simulink model "IceWheel_ControlDesign_Simulink"  (R2021b)
settings: Solver=VariableStepAuto  StartTime=0.0  StopTime=8  RelTol=1e-3
undefined symbols (not defined in the file or in its folder): A, B, C, D, k_m, K_p, T_d, T_motor
libraries: slpidlib x1
settings Model: Creator=elias  LastModifiedBy=SwisensAG
settings SolverCC: AlgebraicLoopSolver=TrustRegion
settings DebuggingCC: SFMachineParentedDataDiag=warning

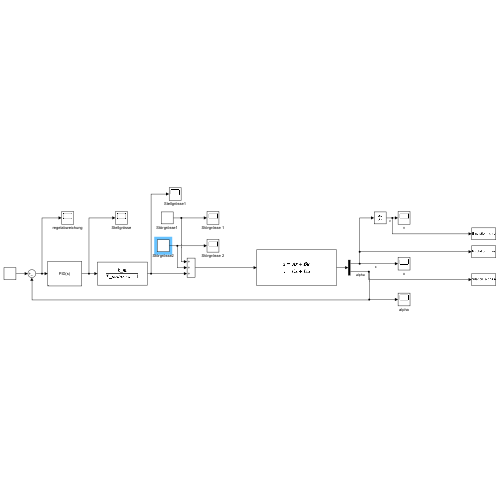
[thumbnail: Simulink's stored preview of the top-level diagram]
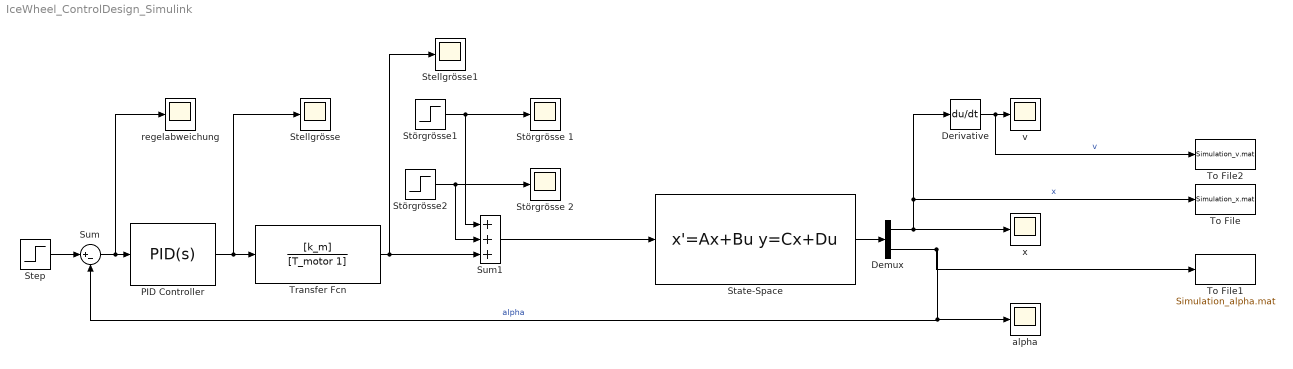
== system IceWheel_ControlDesign_Simulink ==
  Demux : Demux  Outputs=2
  Derivative : Derivative
  PID Controller : slpidlib/PID Controller  Controller=PID  Form=Parallel  TimeDomain=Continuous-time  UseExternalTs=off  SampleTime=-1  IntegratorMethod=Forward Euler  FilterMethod=Forward Euler  ControllerParametersSource=internal  P=K_p  I=2892.84910016522  D=T_d  UseFilter=on  N=1160.80859429286  TunerSelectOption=Transfer Function Based (PID Tuner App)  InitialConditionSource=internal  InitialConditionForIntegrator=0  InitialConditionForFilter=0  DifferentiatorICPrevScaledInput=0  ExternalReset=none  TrackingMode=off  Kt=1  LimitOutput=off  SatLimitsSource=internal  UpperSaturationLimit=inf  LowerSaturationLimit=-inf  LinearizeAsGain=on  AntiWindupMode=none  Kb=1  POutMin=[]  POutMax=[]  IOutMin=[]  IOutMax=[]  DOutMin=[]  DOutMax=[]  NOutMin=[]  NOutMax=[]  SumOutMin=[]  SumOutMax=[]  SaturationOutMin=[]  SaturationOutMax=[]  PParamMin=[]  PParamMax=[]  IParamMin=[]  IParamMax=[]  DParamMin=[]  DParamMax=[]  NParamMin=[]  NParamMax=[]  KbParamMin=[]  KbParamMax=[]  KtParamMin=[]  KtParamMax=[]  KbOutMin=[]  KbOutMax=[]  KtOutMin=[]  KtOutMax=[]  IntegratorOutMin=[]  IntegratorOutMax=[]  FilterOutMin=[]  FilterOutMax=[]  SumI1OutMin=[]  SumI1OutMax=[]  SumI2OutMin=[]  SumI2OutMax=[]  SumI3OutMin=[]  SumI3OutMax=[]  SumI4OutMin=[]  SumI4OutMax=[]  SumDOutMin=[]  SumDOutMax=[]  DifferentiatorOutMin=[]  DifferentiatorOutMax=[]  FilterDiffOutCoefMin=[]  FilterDiffOutCoefMax=[]  ReciprocalOutMin=[]  ReciprocalOutMax=[]  SumDenOutMin=[]  SumDenOutMax=[]  SumNumOutMin=[]  SumNumOutMax=[]  DivideOutMin=[]  DivideOutMax=[]  UdiffTsProdOutMin=[]  UdiffTsProdOutMax=[]  NTsProdOutMin=[]  NTsProdOutMax=[]  UintegralTsProdOutMin=[]  UintegralTsProdOutMax=[]  UngainTsProdOutMin=[]  UngainTsProdOutMax=[]  IntegratorContinuousStateAttributes=''  IntegratorStateMustResolveToSignalObject=off  IntegratorRTWStateStorageClass=Auto  FilterContinuousStateAttributes=''  FilterStateMustResolveToSignalObject=off  FilterRTWStateStorageClass=Auto  ParallelPVariant=InternalParameters  IdealPVariant=Disabled  IVariant=InternalParameters  DVariant=InternalParameters  IntegratorVariant=Continuous  SatVariant=Disabled  AWVariant=Passthrough  PCopyVariant=Disabled  TRVariant=Disabled  FdbkBlocksVariant=Forward  IdealPFdbkVariant=Disabled  SatFdbkVariant=Disabled  DerivativeFilterVariant=ContFilter  NVariant=InternalParameters  NCopyVariant=Disabled  FilterICVariant=InternalICsFilter  IntegratorICVariant=InternalICs  ExternalResetVariant=Disabled  TRSumVariant=Passthrough  SumFdbkVariant=Disabled  SumVariant=Sum_PID  TsampFilterVariant=InternalTs  TsampNgainVariant=Passthrough  TsampIntegralVariant=Passthrough  ExternalSaturationOutDataTypeStr=Inherit: Same as second input
  State-Space : StateSpace  A=A  B=B  C=C  D=D  InitialCondition=[0.1 0 0 0]
  Stellgrösse : Scope
  Stellgrösse1 : Scope
  Step : Step  After=0  SampleTime=0
  Störgrösse 1 : Scope
  Störgrösse 2 : Scope
  Störgrösse1 : Step  After=200  SampleTime=0
  Störgrösse2 : Step  Time=5  After=-500  SampleTime=0
  Sum : Sum  Inputs=|+-
  Sum1 : Sum  Inputs=+++
  To File : ToFile  Filename=Simulation_x.mat  MatrixName=x
      settings: Decimation=4
  To File1 : ToFile  Filename=Simulation_alpha.mat  MatrixName=alpha
      settings: Decimation=4
  To File2 : ToFile  Filename=Simulation_v.mat  MatrixName=v
      settings: Decimation=4
  Transfer Fcn : TransferFcn  Numerator=[k_m]  Denominator=[T_motor 1]
  alpha : Scope
  regelabweichung : Scope
  v : Scope
  x : Scope
  wires:
  Demux/2 -> To File1/1, Sum/2, alpha/1  "alpha"
  State-Space/1 -> Demux/1
  Demux/1 -> To File/1, Derivative/1, x/1  "x"
  Transfer Fcn/1 -> Sum1/3, Stellgrösse1/1
  Step/1 -> Sum/1
  PID Controller/1 -> Stellgrösse/1, Transfer Fcn/1
  Sum/1 -> regelabweichung/1, PID Controller/1
  Derivative/1 -> To File2/1, v/1  "v"
  Sum1/1 -> State-Space/1
  Störgrösse1/1 -> Sum1/1, Störgrösse 1/1
  Störgrösse2/1 -> Sum1/2, Störgrösse 2/1
